simulink model "Tanque"  (R2023b)
settings: Solver=VariableStepAuto  StartTime=0.0  StopTime=10  RelTol=1e-3
values from neighbouring files (symbols this model uses):
  A = [-k1 0; k2 -k3]    [PlotTank.m]
  Ad = sys_d.A    [PlotTank.m]
  B = [1/A1;0]    [PlotTank.m]
  Bd = sys_d.B    [PlotTank.m]
  C = [0 1]    [PlotTank.m]
  Cd = sys_d.C    [PlotTank.m]
  D = [0]    [PlotTank.m]
  Dd = sys_d.D    [PlotTank.m]
  Ts = 0.5    [PlotTank.m]
settings Model: Creator=Shadow  LastModifiedBy=Shadow

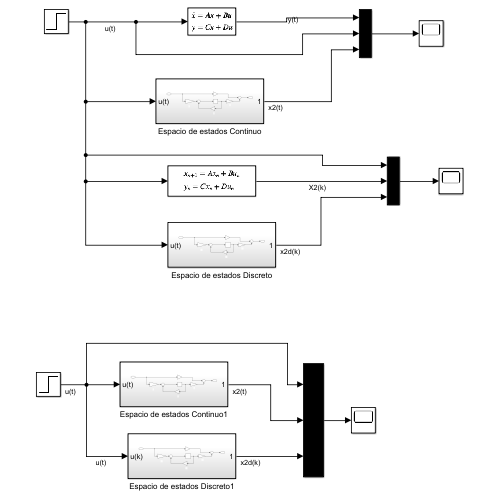
[thumbnail: Simulink's stored preview of the top-level diagram]
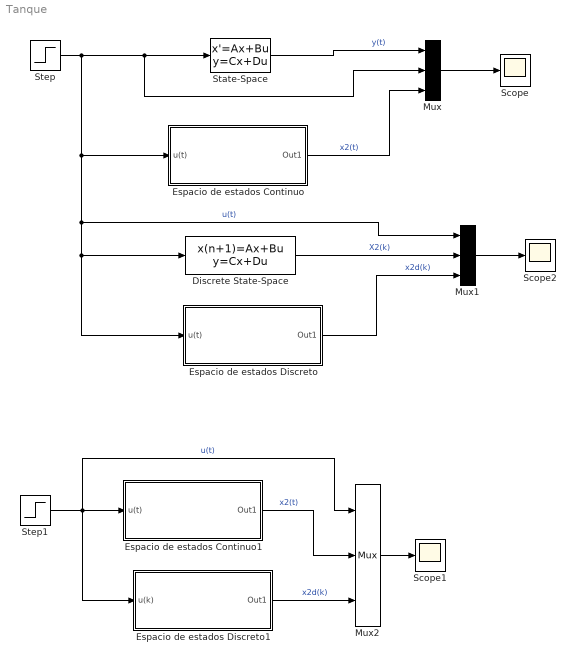
== system Tanque ==
  Discrete State-Space : DiscreteStateSpace  A=Ad  B=Bd  C=Cd  D=Dd  SampleTime=Ts
  Espacio de estados Continuo : Subsystem
  Espacio de estados Continuo1 : Subsystem
  Espacio de estados Discreto : Subsystem
  Espacio de estados Discreto1 : Subsystem
  Mux : Mux  Inputs=3
  Mux1 : Mux  Inputs=3
  Mux2 : Mux  Inputs=3
  Scope : Scope
  Scope1 : Scope
  Scope2 : Scope
  State-Space : StateSpace  A=A  B=B  C=C  D=D  InitialCondition=0
  Step : Step  SampleTime=0
  Step1 : Step  SampleTime=0
  wires:
  Step/1 -> Espacio de estados Continuo/1(u(t)), Mux1/1, Discrete State-Space/1, Espacio de estados Discreto/1(u(t)), Mux/2, State-Space/1  "u(t)"
  State-Space/1 -> Mux/1  "y(t)"
  Mux/1 -> Scope/1
  Espacio de estados Continuo/1(Out1) -> Mux/3  "x2(t)"
  Discrete State-Space/1 -> Mux1/2  "X2(k)"
  Espacio de estados Discreto/1(Out1) -> Mux1/3  "x2d(k)"
  Mux1/1 -> Scope2/1
  Step1/1 -> Espacio de estados Discreto1/1(u(k)), Mux2/1, Espacio de estados Continuo1/1(u(t))  "u(t)"
  Mux2/1 -> Scope1/1
  Espacio de estados Continuo1/1(Out1) -> Mux2/2  "x2(t)"
  Espacio de estados Discreto1/1(Out1) -> Mux2/3  "x2d(k)"

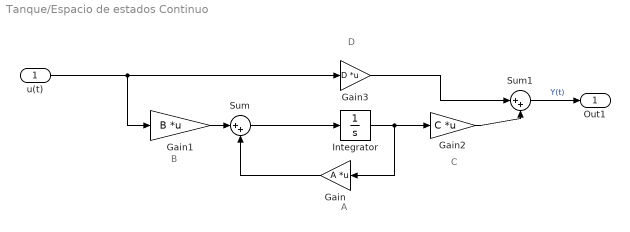
== system Tanque/Espacio de estados Continuo ==
  note: B
  note: C
  note: A
  note: D
  u(t) : Inport
  Gain : Gain  Gain=A  Multiplication=Matrix(K*u)
  Gain1 : Gain  Gain=B  Multiplication=Matrix(K*u) (u vector)
  Gain2 : Gain  Gain=C  Multiplication=Matrix(K*u) (u vector)
  Gain3 : Gain  Gain=D  Multiplication=Matrix(K*u) (u vector)
  Integrator : Integrator
  Sum : Sum  Inputs=|++
  Sum1 : Sum  Inputs=|++
  Out1 : Outport
  wires:
  Sum/1 -> Integrator/1
  Gain/1 -> Sum/2
  Gain1/1 -> Sum/1
  Gain3/1 -> Sum1/1
  Integrator/1 -> Gain2/1, Gain/1
  u(t)/1 -> Gain1/1, Gain3/1
  Sum1/1 -> Out1/1  "Y(t)"
  Gain2/1 -> Sum1/2

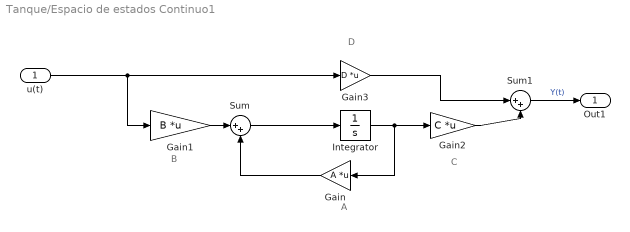
== system Tanque/Espacio de estados Continuo1 ==
  note: D
  note: A
  note: C
  note: B
  u(t) : Inport
  Gain : Gain  Gain=A  Multiplication=Matrix(K*u)
  Gain1 : Gain  Gain=B  Multiplication=Matrix(K*u) (u vector)
  Gain2 : Gain  Gain=C  Multiplication=Matrix(K*u) (u vector)
  Gain3 : Gain  Gain=D  Multiplication=Matrix(K*u) (u vector)
  Integrator : Integrator
  Sum : Sum  Inputs=|++
  Sum1 : Sum  Inputs=|++
  Out1 : Outport
  wires:
  Gain2/1 -> Sum1/2
  Sum1/1 -> Out1/1  "Y(t)"
  u(t)/1 -> Gain3/1, Gain1/1
  Integrator/1 -> Gain/1, Gain2/1
  Gain3/1 -> Sum1/1
  Gain1/1 -> Sum/1
  Gain/1 -> Sum/2
  Sum/1 -> Integrator/1

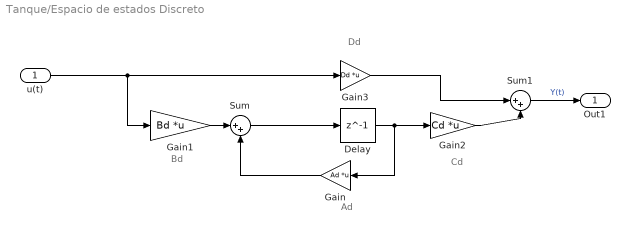
== system Tanque/Espacio de estados Discreto ==
  note: Dd
  note: Ad
  note: Cd
  note: Bd
  u(t) : Inport
  Delay : Delay  DelayLength=1  SampleTime=Ts
  Gain : Gain  Gain=Ad  Multiplication=Matrix(K*u)
  Gain1 : Gain  Gain=Bd  Multiplication=Matrix(K*u) (u vector)
  Gain2 : Gain  Gain=Cd  Multiplication=Matrix(K*u) (u vector)
  Gain3 : Gain  Gain=Dd  Multiplication=Matrix(K*u) (u vector)
  Sum : Sum  Inputs=|++
  Sum1 : Sum  Inputs=|++
  Out1 : Outport
  wires:
  Gain2/1 -> Sum1/2
  Sum1/1 -> Out1/1  "Y(t)"
  u(t)/1 -> Gain3/1, Gain1/1
  Delay/1 -> Gain/1, Gain2/1
  Gain3/1 -> Sum1/1
  Gain1/1 -> Sum/1
  Gain/1 -> Sum/2
  Sum/1 -> Delay/1

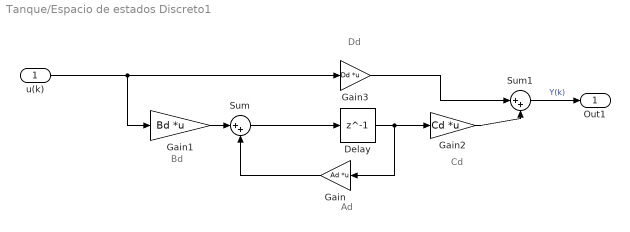
== system Tanque/Espacio de estados Discreto1 ==
  note: Bd
  note: Cd
  note: Ad
  note: Dd
  u(k) : Inport
  Delay : Delay  DelayLength=1  SampleTime=Ts
  Gain : Gain  Gain=Ad  Multiplication=Matrix(K*u)
  Gain1 : Gain  Gain=Bd  Multiplication=Matrix(K*u) (u vector)
  Gain2 : Gain  Gain=Cd  Multiplication=Matrix(K*u) (u vector)
  Gain3 : Gain  Gain=Dd  Multiplication=Matrix(K*u) (u vector)
  Sum : Sum  Inputs=|++
  Sum1 : Sum  Inputs=|++
  Out1 : Outport
  wires:
  Sum/1 -> Delay/1
  Gain/1 -> Sum/2
  Gain1/1 -> Sum/1
  Gain3/1 -> Sum1/1
  Delay/1 -> Gain2/1, Gain/1
  u(k)/1 -> Gain1/1, Gain3/1
  Sum1/1 -> Out1/1  "Y(k)"
  Gain2/1 -> Sum1/2
